simulink model "IdealGen_load_CtrlGen_abc_detailed"  (R2023b)
settings: Solver=VariableStepAuto  StartTime=0.0  StopTime=10  RelTol=1e-3
undefined symbols (not defined in the file): f_nom, H_vsm, Ibase_lv, k_d_vsm, k_p_p_vsm, k_p_q_vsm, ki_q, l_f, L_grid, L_mv, l_t_hvmv, l_t_mvlv, Lbase1v, omega_nom, Pmax, r_f, R_grid, R_mv, r_t_hvmv, r_t_mvlv, Sbase1, Sbase_global, Sbase_t1, Tchange_gfm_ref, Ts, Vbase_hv, Vbase_lv, Vbase_mv, Zbase1v
libraries: spsControlledVoltageSourceLib x6, spsThreePhaseVIMeasurementLib x3, spsPower3phInstantaneousLib x3, spsThreePhaseSeriesRLCBranchLib x3, spsGroundLib x2, spsdq0toabcLib x2, spsThreePhaseTransformerTwoWindingsLib x2, spsThreePhaseSeriesRLCLoadLib x1, spspowerguiLib x1
settings Model: Creator=s183702  LastModifiedBy=s183702

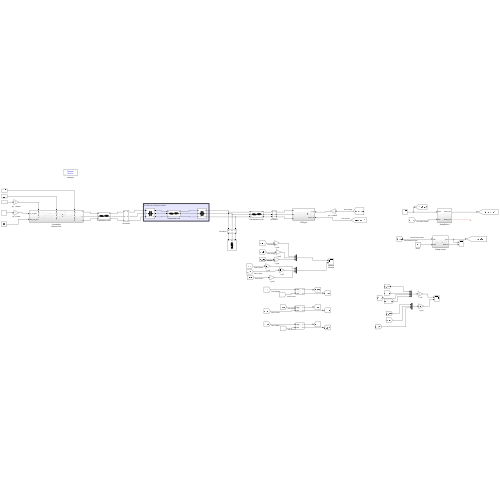
[thumbnail: Simulink's stored preview of the top-level diagram]
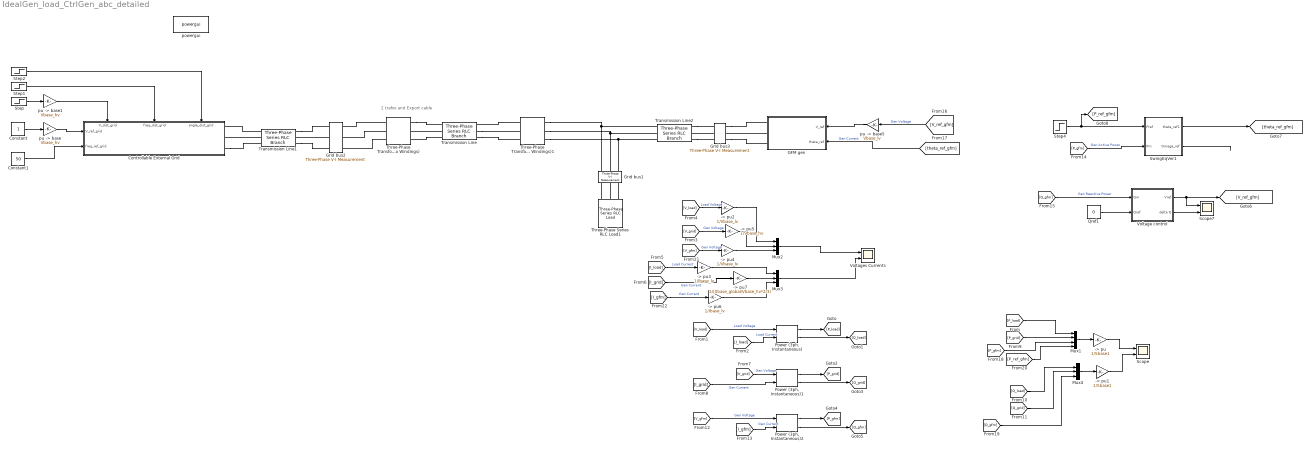
== system IdealGen_load_CtrlGen_abc_detailed ==
  note: 2 trafos and Export cable
  -> pu : Gain  Gain=1/Sbase1
  -> pu1 : Gain  Gain=1/Sbase1
  -> pu2 : Gain  Gain=1/Vbase_lv
  -> pu3 : Gain  Gain=1/Ibase_lv
  -> pu4 : Gain  Gain=1/Vbase_lv
  -> pu5 : Gain  Gain=1/Vbase_hv
  -> pu6 : Gain  Gain=1/Ibase_lv
  -> pu7 : Gain  Gain=1/(Sbase_global/Vbase_hv*2/3)
  Constant : Constant
  Constant1 : Constant  Value=50
  Controllable External Grid : Subsystem
      settings: PortSchema="{\"entries\":[{\"content\":{\"sides\":[{\"content\":{\"connectorIds\":[\"In1\",\"In2\"]},\"type\":\"ConnectorPlacement.EquallySpacedRectSide\",\"uuid\":\"c82e3ee4-47de-4631-9682-a189e406d2fd\"},{\"content\":{\"connectorIds\":[\"RConn1\",\"RConn2\",\"RConn3\"],\"side\":\"RIGHT\"},\"type\":\"ConnectorPlacement.EquallySpacedRectSide\",\"uuid\":\"b806e225-811d-4112-8c3d-45e9b8086e84\"},{\"content\":{\"connectorIds\":[\"In3\",\"In4\",\"In5\"],\"side\":\"TOP\"},\"type\":\"ConnectorPlacement.EquallySpacedRectSide\",\"uuid\":\"c79b677b-bc74-4454-b0f0-10f0f27e0767\"}]},\"type\":\"ConnectorPlacement.EquallySpacedConnector\",\"uuid\":\"44354c03-b4f0-403a-803b-b669dc1296a6\"}],\"packageUris\":[\"http://schema.mathworks.com/mf0/Connector/R2020b\"],\"version\":\"1.0\"}"
  GFM gen : Subsystem
  Grid bus1 : spsThreePhaseVIMeasurementLib/Three-Phase V-I Measurement  VoltageMeasurement=phase-to-ground  SetLabelV=on  LabelV=V_load  Vpu=off  VpuLL=off  CurrentMeasurement=yes  SetLabelI=on  LabelI=I_load  Ipu=off  Pbase=100e6  Vbase=500e3  OutputType=Complex  PhasorSimulation=off  PSBequivalent=0
  Grid bus2 : spsThreePhaseVIMeasurementLib/Three-Phase V-I Measurement  VoltageMeasurement=phase-to-ground  SetLabelV=on  LabelV=V_grid  Vpu=off  VpuLL=off  CurrentMeasurement=yes  SetLabelI=on  LabelI=I_grid  Ipu=off  Pbase=100e6  Vbase=500e3  OutputType=Complex  PhasorSimulation=off  PSBequivalent=0
  Grid bus3 : spsThreePhaseVIMeasurementLib/Three-Phase V-I Measurement  VoltageMeasurement=phase-to-ground  SetLabelV=on  LabelV=V_gfm  Vpu=off  VpuLL=off  CurrentMeasurement=yes  SetLabelI=on  LabelI=I_gfm  Ipu=off  Pbase=100e6  Vbase=500e3  OutputType=Complex  PhasorSimulation=off  PSBequivalent=0
  Mux1 : Mux
  Mux2 : Mux  Inputs=3
  Mux3 : Mux  Inputs=3
  Mux4 : Mux  Inputs=3
  "Power (3ph, Instantaneous)" : spsPower3phInstantaneousLib/Power (3ph, Instantaneous)
  "Power (3ph, Instantaneous)1" : spsPower3phInstantaneousLib/Power (3ph, Instantaneous)
  "Power (3ph, Instantaneous)2" : spsPower3phInstantaneousLib/Power (3ph, Instantaneous)
  Qref1 : Constant  Value=0
  Scope : Scope  NumInputPorts=2
  Scope7 : Scope  NumInputPorts=2
  Step : Step  After=0  SampleTime=0
  Step1 : Step  After=0  SampleTime=0
  Step2 : Step  After=0  SampleTime=0
  Step4 : Step  Time=Tchange_gfm_ref  Before=Sbase1  After=Sbase1*1.2  SampleTime=0
  SwingEqVer1 : Subsystem
  Three-Phase Series RLC Load1 : spsThreePhaseSeriesRLCLoadLib/Three-Phase Series RLC Load  LConnTagsString=A|B|C  Configuration=Y (grounded)  NominalVoltage=Vbase_lv*sqrt(3/2)  Vabc=[1e3 1e3 1e3]  Vabcp=[1e3 1e3 1e3]  NominalFrequency=f_nom  UnbalancedPower=off  ActivePower=Sbase1*0.2  InductivePower=0  CapacitivePower=0  Pabc=[10e3 9e3 11e3]  QLabc=[100 90 110]  QCabc=[100 90 110]  Pabcp=[10e3 9e3 11e3]  QLabcp=[100 90 110]  QCabcp=[100 90 110]  Measurements=None  LoadType=constant PQ
  Three-Phase Transformer (Two Windings) : spsThreePhaseTransformerTwoWindingsLib/Three-Phase Transformer (Two Windings)  Winding1Connection=Yg  Winding2Connection=Yg  CoreType=Three single-phase transformers  SetSaturation=off  Hysteresis=off  DataFile='hysteresis'  SetInitialFlux=off  Measurements=None  UNITS=pu  NominalPower=[ Sbase1 , f_nom ]  Winding1=[ Vbase_hv*sqrt(3/2) , r_t_hvmv/2 , l_t_hvmv/2]  Winding2=[ Vbase_mv*sqrt(3/2) , r_t_hvmv/2, l_t_hvmv/2 ]  Rm=500  Lm=500  L0=0.5  Saturation=[ 0,0 ; 0.0024,1.2 ; 1.0,1.52 ]  InitialFluxes=[ 0.8 , -0.8 , 0.7 ]  BreakLoop=off  DiscreteSolver=Trapezoidal iterative  DataType=off  TransfoNumber=1
  Three-Phase Transformer (Two Windings)1 : spsThreePhaseTransformerTwoWindingsLib/Three-Phase Transformer (Two Windings)  Winding1Connection=Yg  Winding2Connection=Yg  CoreType=Three single-phase transformers  SetSaturation=off  Hysteresis=off  DataFile='hysteresis'  SetInitialFlux=off  Measurements=None  UNITS=pu  NominalPower=[ Sbase_t1 , f_nom ]  Winding1=[ Vbase_mv*sqrt(3/2) , r_t_mvlv/2 , l_t_mvlv/2]  Winding2=[ Vbase_lv*sqrt(3/2) , r_t_mvlv/2, l_t_mvlv/2 ]  Rm=500  Lm=500  L0=0.5  Saturation=[ 0,0 ; 0.0024,1.2 ; 1.0,1.52 ]  InitialFluxes=[ 0.8 , -0.8 , 0.7 ]  BreakLoop=off  DiscreteSolver=Trapezoidal iterative  DataType=off  TransfoNumber=1
  Transmission Line : spsThreePhaseSeriesRLCBranchLib/Three-Phase Series RLC Branch  LConnTagsString=A|B|C  RConnTagsString=A|B|C  BranchType=RL  Resistance=R_mv  Inductance=L_mv  Capacitance=0  Measurements=None
  Transmission Line1 : spsThreePhaseSeriesRLCBranchLib/Three-Phase Series RLC Branch  LConnTagsString=A|B|C  RConnTagsString=A|B|C  BranchType=RL  Resistance=R_grid  Inductance=L_grid  Capacitance=0  Measurements=None
  Transmission Line2 : spsThreePhaseSeriesRLCBranchLib/Three-Phase Series RLC Branch  LConnTagsString=A|B|C  RConnTagsString=A|B|C  BranchType=RL  Resistance=r_f*Zbase1v  Inductance=l_f*Lbase1v  Capacitance=0  Measurements=None
  Voltage control : Subsystem
  Voltages Currents : Scope  NumInputPorts=2
  powergui : spspowerguiLib/powergui  Priority=1  SimulationMode=Discrete  SampleTime=Ts  frequency=60  Iterations=50  frequencyindice=50  Pbase=100e6  ErrMax=1e-4  UnitsV=kV  UnitsW=MW  buscounter=0  FunctionMessages=off  echomessages=off  EnableUseOfTLC=off  CurrentSourceSwitches=off  DisableSnubberDevices=off  DisableRonSwitches=off  DisableVfSwitches=off  DisplayEquations=off  AutomaticDiscreteSolvers=off  SolverType=Tustin/Backward Euler (TBE)  Interpol=off  ExternalGateDelay=off  methode=off  Ts=100  x0status=blocks  SPID=on  SwTol=0  HookPort=off  NonlinearTolerance=1e-4  nMaxIteration=100  ContinueOnMaxIteration=off  RestoreLinks=warning  ResistiveCurrentMeasurement=off  Frange=[0:2:500]  Ylog=off  Xlog=on  ShowGrid=off  save=off  variable=ZData  structure=0  ZoomFFT=off  StartTime=0.0  cycles=1  DisplayStyle=1  fundamental=60  FreqAxis=off  MaxFrequency=1000  frequencyindicesteady=1  RmsSteady=1  display=off
  "pu -> base" : Gain  Gain=Vbase_hv
  "pu -> base1" : Gain  Gain=Vbase_hv
  "pu -> base5" : Gain  Gain=Vbase_lv
  wires:
  [I_load] -> -> pu3/1  "Load Current"
  [V_load] -> -> pu2/1  "Load Voltage"
  [V_grid] -> -> pu5/1  "Gen Voltage"
  [I_grid] -> -> pu7/1  "Gen Current"
  "pu -> base"/1 -> Controllable External Grid/1(V_ref_grid)
  Constant/1 -> "pu -> base"/1
  Constant1/1 -> Controllable External Grid/2(freq_ref_grid)
  Step/1 -> "pu -> base1"/1
  Step1/1 -> Controllable External Grid/4(freq_dist_grid)
  Step2/1 -> Controllable External Grid/5(angle_dist_grid)
  "pu -> base1"/1 -> Controllable External Grid/3(V_dist_grid)
  [V_load] -> "Power (3ph, Instantaneous)"/1  "Load Voltage"
  [I_load] -> "Power (3ph, Instantaneous)"/2  "Load Current"
  [V_grid] -> "Power (3ph, Instantaneous)1"/1  "Gen Voltage"
  [I_grid] -> "Power (3ph, Instantaneous)1"/2  "Gen Current"
  "Power (3ph, Instantaneous)"/1 -> [P_load]
  "Power (3ph, Instantaneous)"/2 -> [Q_load]
  "Power (3ph, Instantaneous)1"/1 -> [P_grid]
  "Power (3ph, Instantaneous)1"/2 -> [Q_grid]
  [Q_load] -> Mux4/1
  [Q_grid] -> Mux4/2
  [P_grid] -> Mux1/2
  [P_load] -> Mux1/1
  Mux4/1 -> -> pu1/1
  Mux1/1 -> -> pu/1
  -> pu/1 -> Scope/1
  -> pu1/1 -> Scope/2
  "pu -> base5"/1 -> GFM gen/1(V_ref)
  "Power (3ph, Instantaneous)2"/2 -> [Q_gfm]
  "Power (3ph, Instantaneous)2"/1 -> [P_gfm]
  [I_gfm] -> "Power (3ph, Instantaneous)2"/2  "Gen Current"
  [V_gfm] -> "Power (3ph, Instantaneous)2"/1  "Gen Voltage"
  Step4/1 -> [P_ref_gfm], SwingEqVer1/1(Pref)
  [P_gfm] -> SwingEqVer1/2(Pm)  "Gen Active Power"
  SwingEqVer1/2(Omega_ref) -> ?
  SwingEqVer1/1(theta_ref1) -> [theta_ref_gfm]
  Qref1/1 -> Voltage control/2(Qref)
  Voltage control/1(Vref) -> Scope7/1, [V_ref_gfm]
  Voltage control/2(delta Q) -> Scope7/2
  [Q_gfm] -> Voltage control/1(Qm)  "Gen Reactive Power"
  [V_ref_gfm] -> "pu -> base5"/1  "Gen Voltage"
  [theta_ref_gfm] -> GFM gen/2(theta_ref)  "Gen Current"
  [P_gfm] -> Mux1/3
  [Q_gfm] -> Mux4/3
  [P_ref_gfm] -> Mux1/4
  [V_gfm] -> -> pu4/1  "Gen Voltage"
  [I_gfm] -> -> pu6/1  "Gen Current"
  Mux2/1 -> Voltages Currents/1
  Mux3/1 -> Voltages Currents/2
  -> pu2/1 -> Mux2/1
  -> pu4/1 -> Mux2/3
  -> pu5/1 -> Mux2/2
  -> pu3/1 -> Mux3/1
  -> pu6/1 -> Mux3/3
  -> pu7/1 -> Mux3/2
  connections:
  Three-Phase Series RLC Load1/LConn1 -- Grid bus1/RConn1
  Three-Phase Series RLC Load1/LConn2 -- Grid bus1/RConn2
  Three-Phase Series RLC Load1/LConn3 -- Grid bus1/RConn3
  Transmission Line2/LConn2 -- Three-Phase Transformer (Two Windings)1/RConn2 -- Grid bus1/LConn2
  Grid bus1/LConn1 -- Three-Phase Transformer (Two Windings)1/RConn1 -- Transmission Line2/LConn1
  Grid bus1/LConn3 -- Three-Phase Transformer (Two Windings)1/RConn3 -- Transmission Line2/LConn3
  Transmission Line1/RConn1 -- Grid bus2/LConn1
  Grid bus2/LConn2 -- Transmission Line1/RConn2
  Transmission Line1/RConn3 -- Grid bus2/LConn3
  Transmission Line1/LConn1 -- Controllable External Grid/RConn1
  Transmission Line1/LConn2 -- Controllable External Grid/RConn2
  Controllable External Grid/RConn3 -- Transmission Line1/LConn3
  GFM gen/RConn2 -- Grid bus3/LConn2
  Grid bus3/LConn1 -- GFM gen/RConn1
  Grid bus3/LConn3 -- GFM gen/RConn3
  Transmission Line2/RConn1 -- Grid bus3/RConn1
  Grid bus3/RConn2 -- Transmission Line2/RConn2
  Transmission Line2/RConn3 -- Grid bus3/RConn3
  Three-Phase Transformer (Two Windings)/LConn2 -- Grid bus2/RConn2
  Three-Phase Transformer (Two Windings)/LConn1 -- Grid bus2/RConn1
  Three-Phase Transformer (Two Windings)/LConn3 -- Grid bus2/RConn3
  Three-Phase Transformer (Two Windings)/RConn1 -- Transmission Line/LConn1
  Transmission Line/LConn2 -- Three-Phase Transformer (Two Windings)/RConn2
  Transmission Line/RConn3 -- Three-Phase Transformer (Two Windings)1/LConn3
  Three-Phase Transformer (Two Windings)1/LConn1 -- Transmission Line/RConn1
  Transmission Line/LConn3 -- Three-Phase Transformer (Two Windings)/RConn3
  Transmission Line/RConn2 -- Three-Phase Transformer (Two Windings)1/LConn2

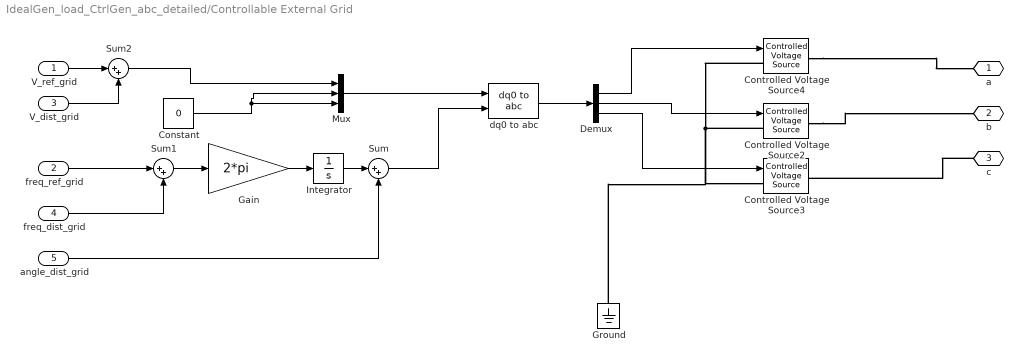
== system IdealGen_load_CtrlGen_abc_detailed/Controllable External Grid ==
  V_ref_grid : Inport
  freq_ref_grid : Inport  Port=2
  V_dist_grid : Inport  Port=3
  freq_dist_grid : Inport  Port=4
  angle_dist_grid : Inport  Port=5
  Constant : Constant  Value=0
  Controlled Voltage Source2 : spsControlledVoltageSourceLib/Controlled Voltage Source  Initialize=on  Source_Type=AC  Amplitude=Vbase_lv*sqrt(2)/sqrt(3)  Phase=-120  Frequency=50  Measurements=None
  Controlled Voltage Source3 : spsControlledVoltageSourceLib/Controlled Voltage Source  Initialize=on  Source_Type=AC  Amplitude=Vbase_lv*sqrt(2)/sqrt(3)  Phase=120  Frequency=50  Measurements=None
  Controlled Voltage Source4 : spsControlledVoltageSourceLib/Controlled Voltage Source  Initialize=on  Source_Type=AC  Amplitude=Vbase_lv*sqrt(2)/sqrt(3)  Phase=0  Frequency=50  Measurements=None
  Demux : Demux  Outputs=3
  Gain : Gain  Gain=2*pi
  Ground : spsGroundLib/Ground  LConnTagsString=a
  Integrator : Integrator
  Mux : Mux  Inputs=3
  Sum : Sum  Inputs=|++
  Sum1 : Sum  Inputs=|++
  Sum2 : Sum  Inputs=|++
  dq0 to abc : spsdq0toabcLib/dq0 to abc  Alignment=Aligned with phase A axis
  a : PMIOPort  Side=Right
  b : PMIOPort  Port=2  Side=Right
  c : PMIOPort  Port=3  Side=Right
  wires:
  Demux/1 -> Controlled Voltage Source4/1
  Demux/2 -> Controlled Voltage Source2/1
  Demux/3 -> Controlled Voltage Source3/1
  Mux/1 -> dq0 to abc/1
  Constant/1 -> Mux/2, Mux/3
  dq0 to abc/1 -> Demux/1
  Sum2/1 -> Mux/1
  Gain/1 -> Integrator/1
  Integrator/1 -> Sum/1
  angle_dist_grid/1 -> Sum/2
  freq_dist_grid/1 -> Sum1/2
  Sum1/1 -> Gain/1
  freq_ref_grid/1 -> Sum1/1
  Sum/1 -> dq0 to abc/2
  V_ref_grid/1 -> Sum2/1
  V_dist_grid/1 -> Sum2/2
  connections:
  Controlled Voltage Source2/LConn1 -- Controlled Voltage Source4/LConn1 -- Ground/LConn1 -- Controlled Voltage Source3/LConn1
  c/RConn1 -- Controlled Voltage Source3/RConn1
  Controlled Voltage Source4/RConn1 -- a/RConn1
  Controlled Voltage Source2/RConn1 -- b/RConn1

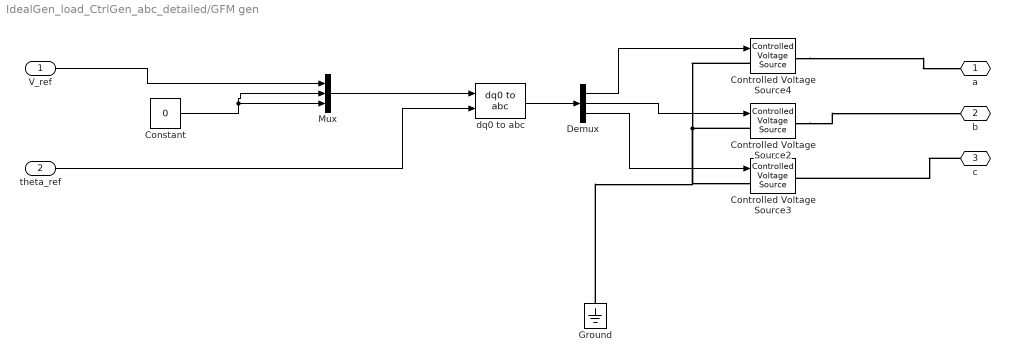
== system IdealGen_load_CtrlGen_abc_detailed/GFM gen ==
  V_ref : Inport
  theta_ref : Inport  Port=2
  Constant : Constant  Value=0
  Controlled Voltage Source2 : spsControlledVoltageSourceLib/Controlled Voltage Source  Initialize=on  Source_Type=AC  Amplitude=Vbase_lv*sqrt(2)/sqrt(3)  Phase=-120  Frequency=50  Measurements=None
  Controlled Voltage Source3 : spsControlledVoltageSourceLib/Controlled Voltage Source  Initialize=on  Source_Type=AC  Amplitude=Vbase_lv*sqrt(2)/sqrt(3)  Phase=120  Frequency=50  Measurements=None
  Controlled Voltage Source4 : spsControlledVoltageSourceLib/Controlled Voltage Source  Initialize=on  Source_Type=AC  Amplitude=Vbase_lv*sqrt(2)/sqrt(3)  Phase=0  Frequency=50  Measurements=None
  Demux : Demux  Outputs=3
  Ground : spsGroundLib/Ground  LConnTagsString=a
  Mux : Mux  Inputs=3
  dq0 to abc : spsdq0toabcLib/dq0 to abc  Alignment=Aligned with phase A axis
  a : PMIOPort  Side=Right
  b : PMIOPort  Port=2  Side=Right
  c : PMIOPort  Port=3  Side=Right
  wires:
  Demux/1 -> Controlled Voltage Source4/1
  Demux/2 -> Controlled Voltage Source2/1
  Demux/3 -> Controlled Voltage Source3/1
  Mux/1 -> dq0 to abc/1
  Constant/1 -> Mux/2, Mux/3
  dq0 to abc/1 -> Demux/1
  V_ref/1 -> Mux/1
  theta_ref/1 -> dq0 to abc/2
  connections:
  Controlled Voltage Source2/LConn1 -- Controlled Voltage Source4/LConn1 -- Ground/LConn1 -- Controlled Voltage Source3/LConn1
  c/RConn1 -- Controlled Voltage Source3/RConn1
  Controlled Voltage Source4/RConn1 -- a/RConn1
  Controlled Voltage Source2/RConn1 -- b/RConn1

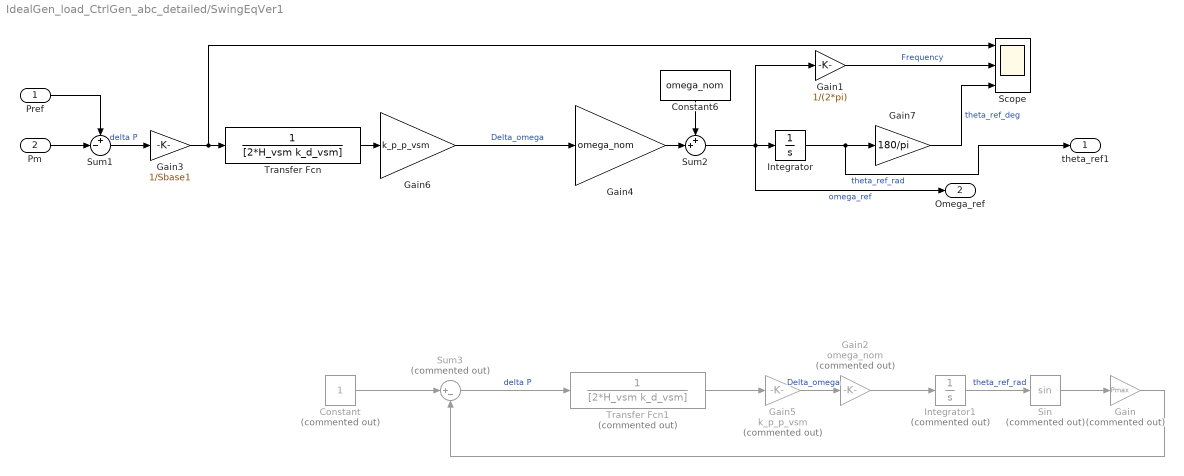
== system IdealGen_load_CtrlGen_abc_detailed/SwingEqVer1 ==
  Pref : Inport
  Pm : Inport  Port=2
  Constant : Constant  Commented=on
  Constant6 : Constant  Value=omega_nom
  Gain : Gain  Commented=on  Gain=Pmax
  Gain1 : Gain  Gain=1/(2*pi)
  Gain2 : Gain  Commented=on  Gain=omega_nom
  Gain3 : Gain  Gain=1/Sbase1
  Gain4 : Gain  Gain=omega_nom
  Gain5 : Gain  Commented=on  Gain=k_p_p_vsm
  Gain6 : Gain  Gain=k_p_p_vsm
  Gain7 : Gain  Gain=180/pi
  Integrator : Integrator  WrappedStateUpperValue=2*pi  WrappedStateLowerValue=0
  Integrator1 : Integrator  Commented=on  WrappedStateUpperValue=2*pi  WrappedStateLowerValue=0
  Scope : Scope  NumInputPorts=3
  Sin : Trigonometry  Commented=on
  Sum1 : Sum  Inputs=+-|
  Sum2 : Sum  Inputs=++|
  Sum3 : Sum  Commented=on  Inputs=|+-
  Transfer Fcn : TransferFcn  Denominator=[2*H_vsm k_d_vsm]
  Transfer Fcn1 : TransferFcn  Commented=on  Denominator=[2*H_vsm k_d_vsm]
  theta_ref1 : Outport
  Omega_ref : Outport  Port=2
  wires:
  Sum1/1 -> Gain3/1  "delta P"
  Integrator/1 -> theta_ref1/1, Gain7/1  "theta_ref_rad"
  Sum2/1 -> Gain1/1, Omega_ref/1, Integrator/1  "omega_ref"
  Transfer Fcn/1 -> Gain6/1
  Gain6/1 -> Gain4/1  "Delta_omega"
  Pm/1 -> Sum1/2
  Gain3/1 -> Scope/1, Transfer Fcn/1
  Gain7/1 -> Scope/3  "theta_ref_deg"
  Pref/1 -> Sum1/1
  Constant6/1 -> Sum2/1
  Gain4/1 -> Sum2/2
  Gain1/1 -> Scope/2  "Frequency"
  Gain5/1 -> Gain2/1  "Delta_omega"
  Transfer Fcn1/1 -> Gain5/1
  Sum3/1 -> Transfer Fcn1/1  "delta P"
  Gain2/1 -> Integrator1/1
  Sin/1 -> Gain/1
  Gain/1 -> Sum3/2
  Constant/1 -> Sum3/1
  Integrator1/1 -> Sin/1  "theta_ref_rad"

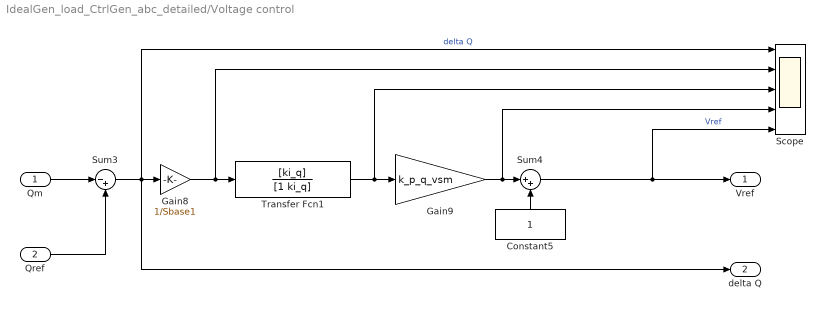
== system IdealGen_load_CtrlGen_abc_detailed/Voltage control ==
  Qm : Inport
  Qref : Inport  Port=2
  Constant5 : Constant
  Gain8 : Gain  Gain=1/Sbase1
  Gain9 : Gain  Gain=k_p_q_vsm
  Scope : Scope  NumInputPorts=5
  Sum3 : Sum  Inputs=|-+
  Sum4 : Sum  Inputs=|++
  Transfer Fcn1 : TransferFcn  Numerator=[ki_q]  Denominator=[1 ki_q]
  Vref : Outport
  delta Q : Outport  Port=2
  wires:
  Constant5/1 -> Sum4/2
  Qm/1 -> Sum3/1
  Gain9/1 -> Scope/4, Sum4/1
  Transfer Fcn1/1 -> Scope/3, Gain9/1
  Gain8/1 -> Scope/2, Transfer Fcn1/1
  Sum3/1 -> Scope/1, delta Q/1, Gain8/1  "delta Q"
  Sum4/1 -> Scope/5, Vref/1  "Vref"
  Qref/1 -> Sum3/2
